simulink model "RCCA_neliniar_releu"  (R2022b)
settings: Solver=FixedStepAuto  StartTime=0.0  StopTime=20  FixedStep=0.01  RelTol=1e-6
values from neighbouring files (symbols this model uses):
  c0 = 5.4698    [script.m]
  ci = 10    [script.m]
  EdR = 49584/8.32    (= 5959.61538462)    [script.m]
  hA = kT*At    (= 18821.555234)    [script.m]
  k0 = 34930800    [script.m]
  mdH = 24953    [script.m]
  q = 10    [script.m]
  rcp = 2093    [script.m]
  T0 = 339.437    [script.m]
  Ti = 38+273    (= 311)    [script.m]
  Tri = 38+273    (= 311)    [script.m]
  V = 10    [script.m]
libraries: slpidlib x2
settings Model: Creator=PS  LastModifiedBy=bn19b
settings SolverCC: ZeroCrossAlgorithm=Adaptive  AlgebraicLoopSolver=TrustRegion
settings DataIOCC: ReturnWorkspaceOutputs=off
settings DebuggingCC: IgnoredZcDiagnostic=none  UnconnectedInputMsg=warning  UnconnectedOutputMsg=warning  UnconnectedLineMsg=warning  SFMachineParentedDataDiag=warning  ArithmeticOperatorsInVariantConditions=warning
settings ModelReferenceCC: EnableRefExpFcnMdlSchedulingChecks=on
settings SFSimCC: SimUseLocalCustomCode=off  CustomCodeUndefinedFunction=UseInterfaceOnly
settings RTWCC: RTWUseLocalCustomCode=off  DLArmComputeVersion=19.05

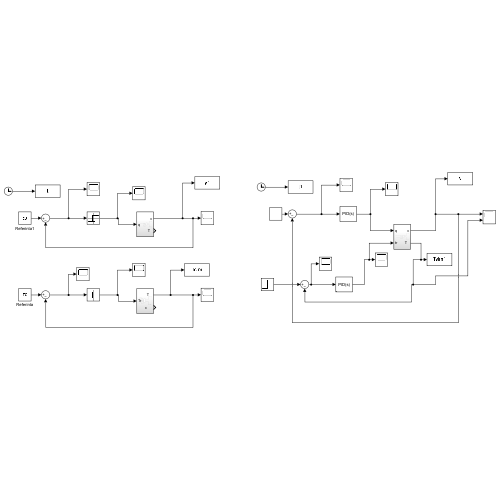
[thumbnail: Simulink's stored preview of the top-level diagram]
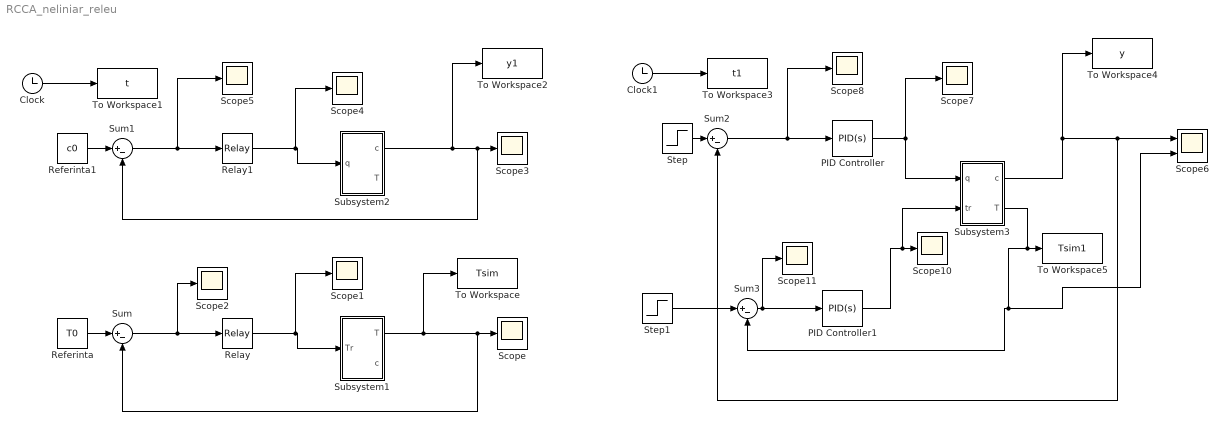
== system RCCA_neliniar_releu ==
  Clock : Clock
  Clock1 : Clock
  PID Controller : slpidlib/PID Controller  Controller=PID  Form=Parallel  TimeDomain=Continuous-time  UseExternalTs=off  SampleTime=-1  IntegratorMethod=Forward Euler  FilterMethod=Forward Euler  ControllerParametersSource=internal  P=13.805  I=17.708  UseKiTs=off  D=0  N=100  UseFilter=on  TunerSelectOption=Transfer Function Based (PID Tuner App)  InitialConditionSource=internal  InitialConditionForIntegrator=q  InitialConditionForFilter=0  DifferentiatorICPrevScaledInput=0  ExternalReset=none  TrackingMode=off  Kt=1  LimitOutput=off  SatLimitsSource=internal  UpperSaturationLimit=inf  LowerSaturationLimit=-inf  LinearizeAsGain=on  AntiWindupMode=none  Kb=1  LimitIntegrator=off  UpperIntegratorSaturationLimit=inf  LowerIntegratorSaturationLimit=-inf  POutMin=[]  POutMax=[]  IOutMin=[]  IOutMax=[]  DOutMin=[]  DOutMax=[]  NOutMin=[]  NOutMax=[]  SumOutMin=[]  SumOutMax=[]  SaturationOutMin=[]  SaturationOutMax=[]  PParamMin=[]  PParamMax=[]  IParamMin=[]  IParamMax=[]  DParamMin=[]  DParamMax=[]  NParamMin=[]  NParamMax=[]  KbParamMin=[]  KbParamMax=[]  KtParamMin=[]  KtParamMax=[]  KbOutMin=[]  KbOutMax=[]  KtOutMin=[]  KtOutMax=[]  IntegratorOutMin=[]  IntegratorOutMax=[]  FilterOutMin=[]  FilterOutMax=[]  SumI1OutMin=[]  SumI1OutMax=[]  SumI2OutMin=[]  SumI2OutMax=[]  SumI3OutMin=[]  SumI3OutMax=[]  SumI4OutMin=[]  SumI4OutMax=[]  SumDOutMin=[]  SumDOutMax=[]  DifferentiatorOutMin=[]  DifferentiatorOutMax=[]  FilterDiffOutCoefMin=[]  FilterDiffOutCoefMax=[]  ReciprocalOutMin=[]  ReciprocalOutMax=[]  SumDenOutMin=[]  SumDenOutMax=[]  SumNumOutMin=[]  SumNumOutMax=[]  DivideOutMin=[]  DivideOutMax=[]  UdiffTsProdOutMin=[]  UdiffTsProdOutMax=[]  NTsProdOutMin=[]  NTsProdOutMax=[]  UintegralTsProdOutMin=[]  UintegralTsProdOutMax=[]  UngainTsProdOutMin=[]  UngainTsProdOutMax=[]  ClampingZeroOutDataTypeStr=Inherit: Inherit via back propagation  ClampingZeroOutMin=[]  ClampingZeroOutMax=[]  FilterDenConstantOutDataTypeStr=Inherit: Inherit via back propagation  FilterDenConstantOutMin=[]  FilterDenConstantOutMax=[]  PCopyOutDataTypeStr=Inherit: Inherit via back propagation  PCopyOutMin=[]  PCopyOutMax=[]  NCopyOutDataTypeStr=Inherit: Inherit via back propagation  NCopyOutMin=[]  NCopyOutMax=[]  IntegratorContinuousStateAttributes=''  IntegratorStateMustResolveToSignalObject=off  IntegratorRTWStateStorageClass=Auto  FilterContinuousStateAttributes=''  FilterStateMustResolveToSignalObject=off  FilterRTWStateStorageClass=Auto  ParallelPVariant=InternalParameters  IdealPVariant=Disabled  IVariant=InternalParameters  DVariant=InternalParameters  IntegratorVariant=Continuous  SatVariant=Disabled  AWVariant=Passthrough  PCopyVariant=Disabled  TRVariant=Disabled  FdbkBlocksVariant=Forward  IdealPFdbkVariant=Disabled  SatFdbkVariant=Disabled  DerivativeFilterVariant=ContFilter  NVariant=InternalParameters  NCopyVariant=Disabled  FilterICVariant=InternalICsFilter  IntegratorICVariant=InternalICs  ExternalResetVariant=Disabled  TRSumVariant=Passthrough  SumFdbkVariant=Disabled  SumVariant=Sum_PID  TsampFilterVariant=InternalTs  TsampNgainVariant=Passthrough  TsampIntegralVariant=Passthrough  ExternalSaturationOutDataTypeStr=Inherit: Same as second input
  PID Controller1 : slpidlib/PID Controller  Controller=PID  Form=Parallel  TimeDomain=Continuous-time  UseExternalTs=off  SampleTime=-1  IntegratorMethod=Forward Euler  FilterMethod=Forward Euler  ControllerParametersSource=internal  P=13.805  I=17.708  UseKiTs=off  D=0  N=100  UseFilter=on  TunerSelectOption=Transfer Function Based (PID Tuner App)  InitialConditionSource=internal  InitialConditionForIntegrator=Tr  InitialConditionForFilter=0  DifferentiatorICPrevScaledInput=0  ExternalReset=none  TrackingMode=off  Kt=1  LimitOutput=off  SatLimitsSource=internal  UpperSaturationLimit=inf  LowerSaturationLimit=-inf  LinearizeAsGain=on  AntiWindupMode=none  Kb=1  LimitIntegrator=off  UpperIntegratorSaturationLimit=inf  LowerIntegratorSaturationLimit=-inf  POutMin=[]  POutMax=[]  IOutMin=[]  IOutMax=[]  DOutMin=[]  DOutMax=[]  NOutMin=[]  NOutMax=[]  SumOutMin=[]  SumOutMax=[]  SaturationOutMin=[]  SaturationOutMax=[]  PParamMin=[]  PParamMax=[]  IParamMin=[]  IParamMax=[]  DParamMin=[]  DParamMax=[]  NParamMin=[]  NParamMax=[]  KbParamMin=[]  KbParamMax=[]  KtParamMin=[]  KtParamMax=[]  KbOutMin=[]  KbOutMax=[]  KtOutMin=[]  KtOutMax=[]  IntegratorOutMin=[]  IntegratorOutMax=[]  FilterOutMin=[]  FilterOutMax=[]  SumI1OutMin=[]  SumI1OutMax=[]  SumI2OutMin=[]  SumI2OutMax=[]  SumI3OutMin=[]  SumI3OutMax=[]  SumI4OutMin=[]  SumI4OutMax=[]  SumDOutMin=[]  SumDOutMax=[]  DifferentiatorOutMin=[]  DifferentiatorOutMax=[]  FilterDiffOutCoefMin=[]  FilterDiffOutCoefMax=[]  ReciprocalOutMin=[]  ReciprocalOutMax=[]  SumDenOutMin=[]  SumDenOutMax=[]  SumNumOutMin=[]  SumNumOutMax=[]  DivideOutMin=[]  DivideOutMax=[]  UdiffTsProdOutMin=[]  UdiffTsProdOutMax=[]  NTsProdOutMin=[]  NTsProdOutMax=[]  UintegralTsProdOutMin=[]  UintegralTsProdOutMax=[]  UngainTsProdOutMin=[]  UngainTsProdOutMax=[]  ClampingZeroOutDataTypeStr=Inherit: Inherit via back propagation  ClampingZeroOutMin=[]  ClampingZeroOutMax=[]  FilterDenConstantOutDataTypeStr=Inherit: Inherit via back propagation  FilterDenConstantOutMin=[]  FilterDenConstantOutMax=[]  PCopyOutDataTypeStr=Inherit: Inherit via back propagation  PCopyOutMin=[]  PCopyOutMax=[]  NCopyOutDataTypeStr=Inherit: Inherit via back propagation  NCopyOutMin=[]  NCopyOutMax=[]  IntegratorContinuousStateAttributes=''  IntegratorStateMustResolveToSignalObject=off  IntegratorRTWStateStorageClass=Auto  FilterContinuousStateAttributes=''  FilterStateMustResolveToSignalObject=off  FilterRTWStateStorageClass=Auto  ParallelPVariant=InternalParameters  IdealPVariant=Disabled  IVariant=InternalParameters  DVariant=InternalParameters  IntegratorVariant=Continuous  SatVariant=Disabled  AWVariant=Passthrough  PCopyVariant=Disabled  TRVariant=Disabled  FdbkBlocksVariant=Forward  IdealPFdbkVariant=Disabled  SatFdbkVariant=Disabled  DerivativeFilterVariant=ContFilter  NVariant=InternalParameters  NCopyVariant=Disabled  FilterICVariant=InternalICsFilter  IntegratorICVariant=InternalICs  ExternalResetVariant=Disabled  TRSumVariant=Passthrough  SumFdbkVariant=Disabled  SumVariant=Sum_PID  TsampFilterVariant=InternalTs  TsampNgainVariant=Passthrough  TsampIntegralVariant=Passthrough  ExternalSaturationOutDataTypeStr=Inherit: Same as second input
  Referinta : Constant  Value=T0
  Referinta1 : Constant  Value=c0
  Relay : Relay  OnSwitchValue=0.1  OffSwitchValue=-0.1  OnOutputValue=Tri+5  OffOutputValue=Tri-5
  Relay1 : Relay  OffSwitchValue=-eps  OnOutputValue=q+2  OffOutputValue=q-2
  Scope{,1..5,7..8,10..11} (10 alike) : Scope
  Scope6 : Scope  NumInputPorts=2
  Step : Step  Time=0  Before=c0  After=c0+0.1  SampleTime=0
  Step1 : Step  Time=0  Before=T0  After=T0+1  SampleTime=0
  Subsystem1 : Subsystem
  Subsystem2 : Subsystem
  Subsystem3 : Subsystem
  Sum{,1..3} (4 alike) : Sum  Inputs=|+-  InputSameDT=on  SaturateOnIntegerOverflow=on  OutDataTypeStr=Inherit: Same as first input
  To Workspace : ToWorkspace  VariableName=Tsim  SampleTime=-1
  To Workspace1 : ToWorkspace  VariableName=t  SampleTime=-1
  To Workspace2 : ToWorkspace  VariableName=y1  SampleTime=-1
  To Workspace3 : ToWorkspace  VariableName=t1  SampleTime=-1
  To Workspace4 : ToWorkspace  VariableName=y  SampleTime=-1
  To Workspace5 : ToWorkspace  VariableName=Tsim1  SampleTime=-1
  wires:
  Sum/1 -> Scope2/1, Relay/1
  Referinta/1 -> Sum/1
  Relay/1 -> Subsystem1/1(Tr), Scope1/1
  Clock/1 -> To Workspace1/1
  Subsystem1/1("T   ") -> Scope/1, Sum/2, To Workspace/1
  Subsystem2/1(c) -> Scope3/1, Sum1/2, To Workspace2/1
  Relay1/1 -> Scope4/1, Subsystem2/1(q)
  Sum1/1 -> Scope5/1, Relay1/1
  Referinta1/1 -> Sum1/1
  Sum2/1 -> PID Controller/1, Scope8/1
  Step/1 -> Sum2/1
  Clock1/1 -> To Workspace3/1
  Subsystem3/1(c) -> Scope6/1, Sum2/2, To Workspace4/1
  PID Controller/1 -> Scope7/1, Subsystem3/1(q)
  Subsystem3/2("T  ") -> Scope6/2, Sum3/2, To Workspace5/1
  Sum3/1 -> PID Controller1/1, Scope11/1
  Step1/1 -> Sum3/1
  PID Controller1/1 -> Subsystem3/2(tr), Scope10/1

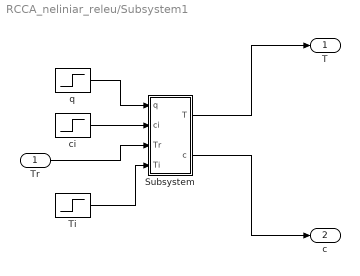
== system RCCA_neliniar_releu/Subsystem1 ==
  Tr : Inport
  Subsystem : Subsystem
  Ti : Step  Time=0  Before=Ti  After=Ti  SampleTime=0
  ci : Step  Time=0  Before=ci  After=ci  SampleTime=0
  "q  " : Step  Time=0  Before=q  After=q  SampleTime=0
  "T   " : Outport
  "c     " : Outport  Port=2
  wires:
  "q  "/1 -> Subsystem/1(q)
  ci/1 -> Subsystem/2(ci)
  Ti/1 -> Subsystem/4(Ti)
  Tr/1 -> Subsystem/3(Tr)
  Subsystem/2("c   ") -> "c     "/1
  Subsystem/1("T  ") -> "T   "/1

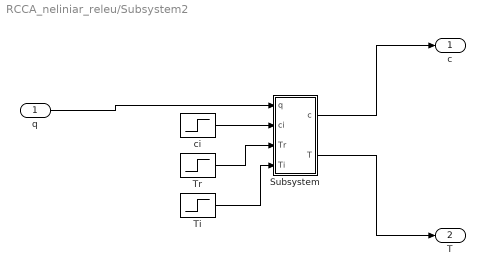
== system RCCA_neliniar_releu/Subsystem2 ==
  q : Inport
  Subsystem : Subsystem
  Ti : Step  Time=0  Before=Ti  After=Ti  SampleTime=0
  Tr : Step  Time=0  Before=Tri  After=Tri  SampleTime=0
  ci : Step  Time=0  Before=ci  After=ci  SampleTime=0
  c : Outport
  "T  " : Outport  Port=2
  wires:
  q/1 -> Subsystem/1(q)
  ci/1 -> Subsystem/2(ci)
  Ti/1 -> Subsystem/4(Ti)
  Tr/1 -> Subsystem/3(Tr)
  Subsystem/2("T  ") -> "T  "/1
  Subsystem/1(c) -> c/1

== system RCCA_neliniar_releu/Subsystem3 ==
  q : Inport
  tr : Inport  Port=2
  Subsystem : Subsystem
  Ti : Step  Time=0  Before=Ti  After=Ti  SampleTime=0
  ci : Step  Time=0  Before=ci  After=ci  SampleTime=0
  c : Outport
  "T  " : Outport  Port=2
  wires:
  q/1 -> Subsystem/1(q)
  ci/1 -> Subsystem/2(ci)
  Ti/1 -> Subsystem/4(Ti)
  tr/1 -> Subsystem/3(Tr)
  Subsystem/2("T  ") -> "T  "/1
  Subsystem/1(c) -> c/1

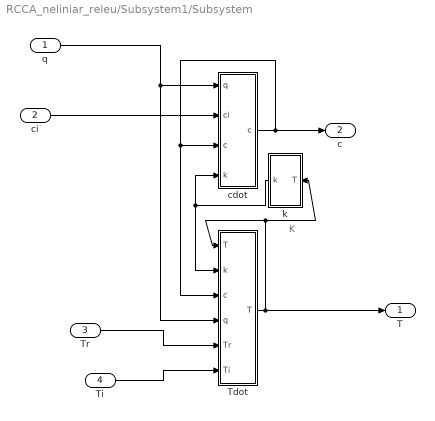
== system RCCA_neliniar_releu/Subsystem1/Subsystem ==
  note: K
  q : Inport
  ci : Inport  Port=2
  Tr : Inport  Port=3
  Ti : Inport  Port=4
  Tdot : Subsystem
  cdot : Subsystem
  k : Subsystem
  "T  " : Outport
  "c   " : Outport  Port=2
  wires:
  Tdot/1("T  ") -> "T  "/1, k/1(T), Tdot/1(T)
  k/1(k) -> Tdot/2(k), cdot/4(k)
  cdot/1(c) -> "c   "/1, cdot/3("c  "), Tdot/3(c)
  q/1 -> cdot/1(q), Tdot/4(q)
  Ti/1 -> Tdot/6(Ti)
  ci/1 -> cdot/2(ci)
  Tr/1 -> Tdot/5(Tr)

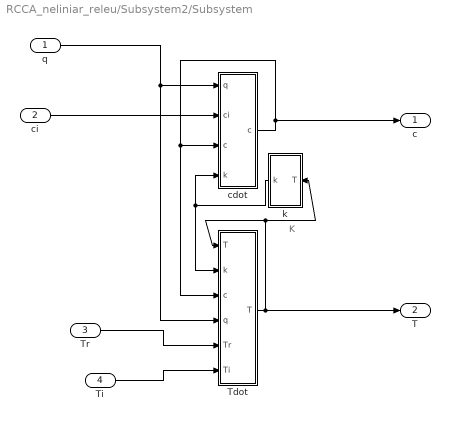
== system RCCA_neliniar_releu/Subsystem2/Subsystem ==
  note: K
  q : Inport
  ci : Inport  Port=2
  Tr : Inport  Port=3
  Ti : Inport  Port=4
  Tdot : Subsystem
  cdot : Subsystem
  k : Subsystem
  c : Outport
  "T  " : Outport  Port=2
  wires:
  Tdot/1("T  ") -> "T  "/1, k/1(T), Tdot/1(T)
  k/1(k) -> Tdot/2(k), cdot/4(k)
  cdot/1(c) -> c/1, cdot/3("c  "), Tdot/3(c)
  q/1 -> cdot/1(q), Tdot/4(q)
  Ti/1 -> Tdot/6(Ti)
  ci/1 -> cdot/2(ci)
  Tr/1 -> Tdot/5(Tr)

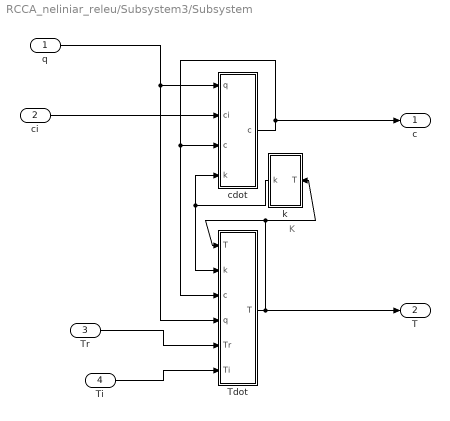
== system RCCA_neliniar_releu/Subsystem3/Subsystem ==
  note: K
  q : Inport
  ci : Inport  Port=2
  Tr : Inport  Port=3
  Ti : Inport  Port=4
  Tdot : Subsystem
  cdot : Subsystem
  k : Subsystem
  c : Outport
  "T  " : Outport  Port=2
  wires:
  Tdot/1("T  ") -> "T  "/1, k/1(T), Tdot/1(T)
  k/1(k) -> Tdot/2(k), cdot/4(k)
  cdot/1(c) -> c/1, cdot/3("c  "), Tdot/3(c)
  q/1 -> cdot/1(q), Tdot/4(q)
  Ti/1 -> Tdot/6(Ti)
  ci/1 -> cdot/2(ci)
  Tr/1 -> Tdot/5(Tr)

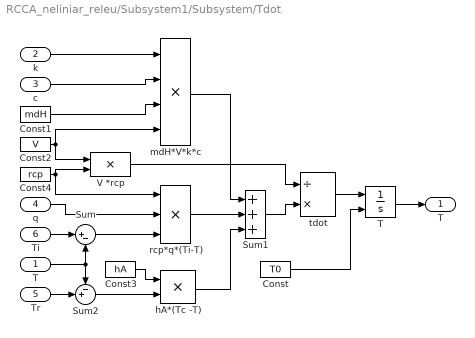
== system RCCA_neliniar_releu/Subsystem1/Subsystem/Tdot ==
  T : Inport  Interpolate=off
  k : Inport  Port=2  Interpolate=off
  c : Inport  Port=3  Interpolate=off
  q : Inport  Port=4  Interpolate=off
  Tr : Inport  Port=5  Interpolate=off
  Ti : Inport  Port=6  Interpolate=off
  Const : Constant  Value=T0
  Const1 : Constant  Value=mdH
  Const2 : Constant  Value=V
  Const3 : Constant  Value=hA
  Const4 : Constant  Value=rcp
  Sum : Sum  Inputs=|+-  InputSameDT=on  SaturateOnIntegerOverflow=on  OutDataTypeStr=Inherit: Same as first input
  Sum1 : Sum  Inputs=+++  InputSameDT=on  SaturateOnIntegerOverflow=on  OutDataTypeStr=Inherit: Same as first input
  Sum2 : Sum  Inputs=-+|  InputSameDT=on  SaturateOnIntegerOverflow=on  OutDataTypeStr=Inherit: Same as first input
  "T " : Integrator  InitialConditionSource=external
  V *rcp : Product  Inputs=**  InputSameDT=on  RndMeth=Zero  SaturateOnIntegerOverflow=on  OutDataTypeStr=Inherit: Same as first input
  hA*(Tc -T) : Product  Inputs=**  InputSameDT=on  RndMeth=Zero  SaturateOnIntegerOverflow=on  OutDataTypeStr=Inherit: Same as first input
  mdH*V*k*c : Product  Inputs=****  InputSameDT=on  RndMeth=Zero  SaturateOnIntegerOverflow=on  OutDataTypeStr=Inherit: Same as first input
  rcp*q*(Ti-T) : Product  Inputs=***  InputSameDT=on  RndMeth=Zero  SaturateOnIntegerOverflow=on  OutDataTypeStr=Inherit: Same as first input
  tdot : Product  Inputs=/*  InputSameDT=on  RndMeth=Zero  SaturateOnIntegerOverflow=on  OutDataTypeStr=Inherit: Same as first input
  "T  " : Outport
  wires:
  Ti/1 -> Sum/1
  Sum/1 -> rcp*q*(Ti-T)/3
  q/1 -> rcp*q*(Ti-T)/2
  T/1 -> Sum/2, Sum2/1
  Tr/1 -> Sum2/2
  Sum2/1 -> hA*(Tc -T)/2
  Const3/1 -> hA*(Tc -T)/1
  k/1 -> mdH*V*k*c/1
  c/1 -> mdH*V*k*c/2
  Const1/1 -> mdH*V*k*c/3
  mdH*V*k*c/1 -> Sum1/1
  rcp*q*(Ti-T)/1 -> Sum1/2
  hA*(Tc -T)/1 -> Sum1/3
  Const2/1 -> mdH*V*k*c/4, V *rcp/1
  Const4/1 -> rcp*q*(Ti-T)/1, V *rcp/2
  V *rcp/1 -> tdot/1
  Sum1/1 -> tdot/2
  tdot/1 -> "T "/1
  Const/1 -> "T "/2
  "T "/1 -> "T  "/1

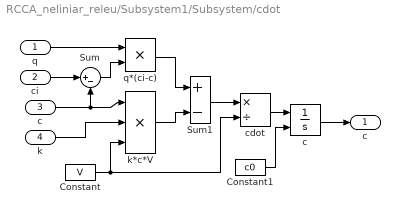
== system RCCA_neliniar_releu/Subsystem1/Subsystem/cdot ==
  q : Inport  Interpolate=off
  ci : Inport  Port=2  Interpolate=off
  "c  " : Inport  Port=3  Interpolate=off
  k : Inport  Port=4  Interpolate=off
  Constant : Constant  Value=V
  Constant1 : Constant  Value=c0
  Sum : Sum  Inputs=|+-  InputSameDT=on  SaturateOnIntegerOverflow=on  OutDataTypeStr=Inherit: Same as first input
  Sum1 : Sum  Inputs=+-  InputSameDT=on  SaturateOnIntegerOverflow=on  OutDataTypeStr=Inherit: Same as first input
  "c " : Integrator  InitialConditionSource=external
  cdot : Product  Inputs=*/  InputSameDT=on  RndMeth=Zero  SaturateOnIntegerOverflow=on  OutDataTypeStr=Inherit: Same as first input
  k*c*V : Product  Inputs=***  InputSameDT=on  RndMeth=Zero  SaturateOnIntegerOverflow=on  OutDataTypeStr=Inherit: Same as first input
  q*(ci-c) : Product  Inputs=**  InputSameDT=on  RndMeth=Zero  SaturateOnIntegerOverflow=on  OutDataTypeStr=Inherit: Same as first input
  c : Outport
  wires:
  ci/1 -> Sum/1
  "c  "/1 -> k*c*V/1, Sum/2
  q/1 -> q*(ci-c)/1
  Sum/1 -> q*(ci-c)/2
  k/1 -> k*c*V/2
  q*(ci-c)/1 -> Sum1/1
  k*c*V/1 -> Sum1/2
  Sum1/1 -> cdot/1
  Constant/1 -> k*c*V/3, cdot/2
  cdot/1 -> "c "/1
  "c "/1 -> c/1
  Constant1/1 -> "c "/2

== system RCCA_neliniar_releu/Subsystem1/Subsystem/k ==
  T : Inport  Interpolate=off
  Const : Constant  Value=-EdR
  Const1 : Constant  Value=k0
  M Fcn : Math  SignedPower=on
  Product : Product  Inputs=*/  InputSameDT=on  RndMeth=Zero  SaturateOnIntegerOverflow=on  OutDataTypeStr=Inherit: Same as first input
  Product1 : Product  Inputs=**  InputSameDT=on  RndMeth=Zero  SaturateOnIntegerOverflow=on  OutDataTypeStr=Inherit: Same as first input
  k : Outport
  wires:
  Const/1 -> Product/1
  T/1 -> Product/2
  Product/1 -> M Fcn/1
  M Fcn/1 -> Product1/1
  Const1/1 -> Product1/2
  Product1/1 -> k/1

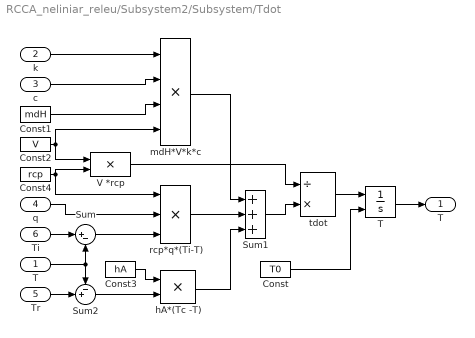
== system RCCA_neliniar_releu/Subsystem2/Subsystem/Tdot ==
  T : Inport  Interpolate=off
  k : Inport  Port=2  Interpolate=off
  c : Inport  Port=3  Interpolate=off
  q : Inport  Port=4  Interpolate=off
  Tr : Inport  Port=5  Interpolate=off
  Ti : Inport  Port=6  Interpolate=off
  Const : Constant  Value=T0
  Const1 : Constant  Value=mdH
  Const2 : Constant  Value=V
  Const3 : Constant  Value=hA
  Const4 : Constant  Value=rcp
  Sum : Sum  Inputs=|+-  InputSameDT=on  SaturateOnIntegerOverflow=on  OutDataTypeStr=Inherit: Same as first input
  Sum1 : Sum  Inputs=+++  InputSameDT=on  SaturateOnIntegerOverflow=on  OutDataTypeStr=Inherit: Same as first input
  Sum2 : Sum  Inputs=-+|  InputSameDT=on  SaturateOnIntegerOverflow=on  OutDataTypeStr=Inherit: Same as first input
  "T " : Integrator  InitialConditionSource=external
  V *rcp : Product  Inputs=**  InputSameDT=on  RndMeth=Zero  SaturateOnIntegerOverflow=on  OutDataTypeStr=Inherit: Same as first input
  hA*(Tc -T) : Product  Inputs=**  InputSameDT=on  RndMeth=Zero  SaturateOnIntegerOverflow=on  OutDataTypeStr=Inherit: Same as first input
  mdH*V*k*c : Product  Inputs=****  InputSameDT=on  RndMeth=Zero  SaturateOnIntegerOverflow=on  OutDataTypeStr=Inherit: Same as first input
  rcp*q*(Ti-T) : Product  Inputs=***  InputSameDT=on  RndMeth=Zero  SaturateOnIntegerOverflow=on  OutDataTypeStr=Inherit: Same as first input
  tdot : Product  Inputs=/*  InputSameDT=on  RndMeth=Zero  SaturateOnIntegerOverflow=on  OutDataTypeStr=Inherit: Same as first input
  "T  " : Outport
  wires:
  Ti/1 -> Sum/1
  Sum/1 -> rcp*q*(Ti-T)/3
  q/1 -> rcp*q*(Ti-T)/2
  T/1 -> Sum/2, Sum2/1
  Tr/1 -> Sum2/2
  Sum2/1 -> hA*(Tc -T)/2
  Const3/1 -> hA*(Tc -T)/1
  k/1 -> mdH*V*k*c/1
  c/1 -> mdH*V*k*c/2
  Const1/1 -> mdH*V*k*c/3
  mdH*V*k*c/1 -> Sum1/1
  rcp*q*(Ti-T)/1 -> Sum1/2
  hA*(Tc -T)/1 -> Sum1/3
  Const2/1 -> mdH*V*k*c/4, V *rcp/1
  Const4/1 -> rcp*q*(Ti-T)/1, V *rcp/2
  V *rcp/1 -> tdot/1
  Sum1/1 -> tdot/2
  tdot/1 -> "T "/1
  Const/1 -> "T "/2
  "T "/1 -> "T  "/1

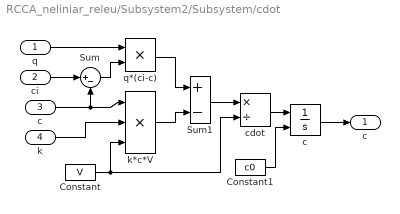
== system RCCA_neliniar_releu/Subsystem2/Subsystem/cdot ==
  q : Inport  Interpolate=off
  ci : Inport  Port=2  Interpolate=off
  "c  " : Inport  Port=3  Interpolate=off
  k : Inport  Port=4  Interpolate=off
  Constant : Constant  Value=V
  Constant1 : Constant  Value=c0
  Sum : Sum  Inputs=|+-  InputSameDT=on  SaturateOnIntegerOverflow=on  OutDataTypeStr=Inherit: Same as first input
  Sum1 : Sum  Inputs=+-  InputSameDT=on  SaturateOnIntegerOverflow=on  OutDataTypeStr=Inherit: Same as first input
  "c " : Integrator  InitialConditionSource=external
  cdot : Product  Inputs=*/  InputSameDT=on  RndMeth=Zero  SaturateOnIntegerOverflow=on  OutDataTypeStr=Inherit: Same as first input
  k*c*V : Product  Inputs=***  InputSameDT=on  RndMeth=Zero  SaturateOnIntegerOverflow=on  OutDataTypeStr=Inherit: Same as first input
  q*(ci-c) : Product  Inputs=**  InputSameDT=on  RndMeth=Zero  SaturateOnIntegerOverflow=on  OutDataTypeStr=Inherit: Same as first input
  c : Outport
  wires:
  ci/1 -> Sum/1
  "c  "/1 -> k*c*V/1, Sum/2
  q/1 -> q*(ci-c)/1
  Sum/1 -> q*(ci-c)/2
  k/1 -> k*c*V/2
  q*(ci-c)/1 -> Sum1/1
  k*c*V/1 -> Sum1/2
  Sum1/1 -> cdot/1
  Constant/1 -> k*c*V/3, cdot/2
  cdot/1 -> "c "/1
  "c "/1 -> c/1
  Constant1/1 -> "c "/2

== system RCCA_neliniar_releu/Subsystem2/Subsystem/k ==
  T : Inport  Interpolate=off
  Const : Constant  Value=-EdR
  Const1 : Constant  Value=k0
  M Fcn : Math  SignedPower=on
  Product : Product  Inputs=*/  InputSameDT=on  RndMeth=Zero  SaturateOnIntegerOverflow=on  OutDataTypeStr=Inherit: Same as first input
  Product1 : Product  Inputs=**  InputSameDT=on  RndMeth=Zero  SaturateOnIntegerOverflow=on  OutDataTypeStr=Inherit: Same as first input
  k : Outport
  wires:
  Const/1 -> Product/1
  T/1 -> Product/2
  Product/1 -> M Fcn/1
  M Fcn/1 -> Product1/1
  Const1/1 -> Product1/2
  Product1/1 -> k/1

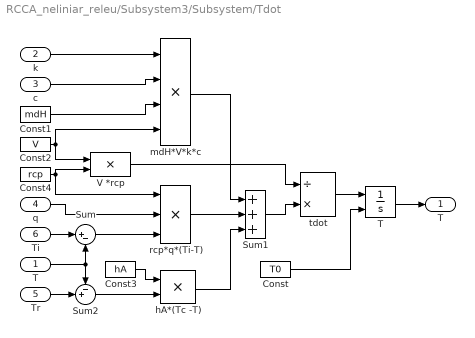
== system RCCA_neliniar_releu/Subsystem3/Subsystem/Tdot ==
  T : Inport  Interpolate=off
  k : Inport  Port=2  Interpolate=off
  c : Inport  Port=3  Interpolate=off
  q : Inport  Port=4  Interpolate=off
  Tr : Inport  Port=5  Interpolate=off
  Ti : Inport  Port=6  Interpolate=off
  Const : Constant  Value=T0
  Const1 : Constant  Value=mdH
  Const2 : Constant  Value=V
  Const3 : Constant  Value=hA
  Const4 : Constant  Value=rcp
  Sum : Sum  Inputs=|+-  InputSameDT=on  SaturateOnIntegerOverflow=on  OutDataTypeStr=Inherit: Same as first input
  Sum1 : Sum  Inputs=+++  InputSameDT=on  SaturateOnIntegerOverflow=on  OutDataTypeStr=Inherit: Same as first input
  Sum2 : Sum  Inputs=-+|  InputSameDT=on  SaturateOnIntegerOverflow=on  OutDataTypeStr=Inherit: Same as first input
  "T " : Integrator  InitialConditionSource=external
  V *rcp : Product  Inputs=**  InputSameDT=on  RndMeth=Zero  SaturateOnIntegerOverflow=on  OutDataTypeStr=Inherit: Same as first input
  hA*(Tc -T) : Product  Inputs=**  InputSameDT=on  RndMeth=Zero  SaturateOnIntegerOverflow=on  OutDataTypeStr=Inherit: Same as first input
  mdH*V*k*c : Product  Inputs=****  InputSameDT=on  RndMeth=Zero  SaturateOnIntegerOverflow=on  OutDataTypeStr=Inherit: Same as first input
  rcp*q*(Ti-T) : Product  Inputs=***  InputSameDT=on  RndMeth=Zero  SaturateOnIntegerOverflow=on  OutDataTypeStr=Inherit: Same as first input
  tdot : Product  Inputs=/*  InputSameDT=on  RndMeth=Zero  SaturateOnIntegerOverflow=on  OutDataTypeStr=Inherit: Same as first input
  "T  " : Outport
  wires:
  Ti/1 -> Sum/1
  Sum/1 -> rcp*q*(Ti-T)/3
  q/1 -> rcp*q*(Ti-T)/2
  T/1 -> Sum/2, Sum2/1
  Tr/1 -> Sum2/2
  Sum2/1 -> hA*(Tc -T)/2
  Const3/1 -> hA*(Tc -T)/1
  k/1 -> mdH*V*k*c/1
  c/1 -> mdH*V*k*c/2
  Const1/1 -> mdH*V*k*c/3
  mdH*V*k*c/1 -> Sum1/1
  rcp*q*(Ti-T)/1 -> Sum1/2
  hA*(Tc -T)/1 -> Sum1/3
  Const2/1 -> mdH*V*k*c/4, V *rcp/1
  Const4/1 -> rcp*q*(Ti-T)/1, V *rcp/2
  V *rcp/1 -> tdot/1
  Sum1/1 -> tdot/2
  tdot/1 -> "T "/1
  Const/1 -> "T "/2
  "T "/1 -> "T  "/1

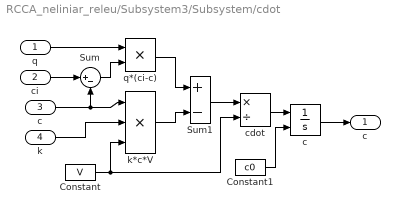
== system RCCA_neliniar_releu/Subsystem3/Subsystem/cdot ==
  q : Inport  Interpolate=off
  ci : Inport  Port=2  Interpolate=off
  "c  " : Inport  Port=3  Interpolate=off
  k : Inport  Port=4  Interpolate=off
  Constant : Constant  Value=V
  Constant1 : Constant  Value=c0
  Sum : Sum  Inputs=|+-  InputSameDT=on  SaturateOnIntegerOverflow=on  OutDataTypeStr=Inherit: Same as first input
  Sum1 : Sum  Inputs=+-  InputSameDT=on  SaturateOnIntegerOverflow=on  OutDataTypeStr=Inherit: Same as first input
  "c " : Integrator  InitialConditionSource=external
  cdot : Product  Inputs=*/  InputSameDT=on  RndMeth=Zero  SaturateOnIntegerOverflow=on  OutDataTypeStr=Inherit: Same as first input
  k*c*V : Product  Inputs=***  InputSameDT=on  RndMeth=Zero  SaturateOnIntegerOverflow=on  OutDataTypeStr=Inherit: Same as first input
  q*(ci-c) : Product  Inputs=**  InputSameDT=on  RndMeth=Zero  SaturateOnIntegerOverflow=on  OutDataTypeStr=Inherit: Same as first input
  c : Outport
  wires:
  ci/1 -> Sum/1
  "c  "/1 -> k*c*V/1, Sum/2
  q/1 -> q*(ci-c)/1
  Sum/1 -> q*(ci-c)/2
  k/1 -> k*c*V/2
  q*(ci-c)/1 -> Sum1/1
  k*c*V/1 -> Sum1/2
  Sum1/1 -> cdot/1
  Constant/1 -> k*c*V/3, cdot/2
  cdot/1 -> "c "/1
  "c "/1 -> c/1
  Constant1/1 -> "c "/2

== system RCCA_neliniar_releu/Subsystem3/Subsystem/k ==
  T : Inport  Interpolate=off
  Const : Constant  Value=-EdR
  Const1 : Constant  Value=k0
  M Fcn : Math  SignedPower=on
  Product : Product  Inputs=*/  InputSameDT=on  RndMeth=Zero  SaturateOnIntegerOverflow=on  OutDataTypeStr=Inherit: Same as first input
  Product1 : Product  Inputs=**  InputSameDT=on  RndMeth=Zero  SaturateOnIntegerOverflow=on  OutDataTypeStr=Inherit: Same as first input
  k : Outport
  wires:
  Const/1 -> Product/1
  T/1 -> Product/2
  Product/1 -> M Fcn/1
  M Fcn/1 -> Product1/1
  Const1/1 -> Product1/2
  Product1/1 -> k/1
